simulink library "Pump_Lib"  (R2014a)
settings: Solver=ode45  StartTime=0.0  StopTime=10.0  RelTol=1e-3
undefined symbols (not defined in the file): APN_Param
libraries: Pump_Lib x3, powerlib x3
Description:
  | Copyright 2014 The MathWorks, Inc.
settings Model: Creator=smiller  LastModifiedBy=psanghvi

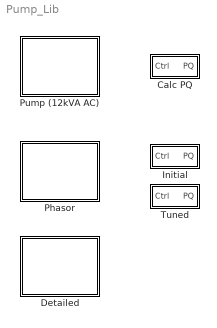
== system Pump_Lib ==
  Calc PQ : Subsystem  BlockChoice=Initial
      settings: TemplateBlock=self  MemberBlocks=Initial,Tuned
  Detailed : Subsystem
      mask Display: image(imread('PumpAC_Detailed_IMAGE.jpg'));
  Initial : Subsystem
  Phasor : Subsystem
      mask Display: image(imread('PumpAC_Phasor_IMAGE.jpg'));
  Pump (12kVA AC) : Subsystem  BlockChoice=Detailed
      settings: TemplateBlock=self  MemberBlocks=Detailed,Phasor
  Tuned : Subsystem

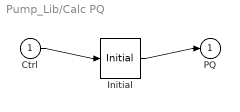
== system Pump_Lib/Calc PQ ==
  Ctrl : Inport
  Initial : Pump_Lib/Initial
  PQ : Outport
  wires:
  Ctrl/1 -> Initial/1
  Initial/1 -> PQ/1

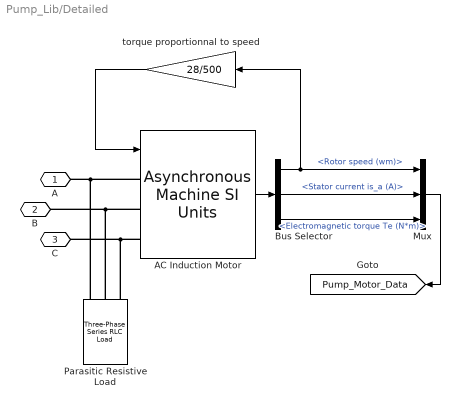
== system Pump_Lib/Detailed ==
  AC Induction Motor : powerlib/Machines/Asynchronous Machine SI Units  PresetModel=No  MechanicalLoad=Torque Tm  ShowDetailedParameters=on  RotorType=Squirrel-cage  ReferenceFrame=Rotor  Units=SI  MeasurementBus=off  NominalParameters=[12e3 200 400]  Stator=[0.2761 0.002191/10]  Rotor=[0.16 0.002191/10]  Cage1=[ 0.022 0.226/377]  Cage2=[ 0.022 0.226/377]  Lm=0.07614  Mechanical=[0.01 0 8]  PolePairs=8  InitialConditions=[0 0 0.850924 0.850924 0.850924 -89.9171 -209.917 30.0829]*0+[0,0 0,0,0 0,0,0]  SimulateSaturation=off  Saturation=[14.03593122, 27.81365428, 53.79336849, 72.68890987, 97.98006896, 148.6815601, 215.7428561, 302.9841135, 428.7778367 ; 230, 322, 414, 460, 506, 552, 598, 644, 690]  LoadFlowParameters=0  TsPowergui=0  TsBlock=-1  IterativeModel=Forward Euler  Pmec=0
  Bus Selector : BusSelector  OutputSignals=Mechanical.Rotor speed (wm),Stator measurements.Stator current is_a (A),Mechanical.Electromagnetic torque Te (N*m)
  Mux : Mux  Inputs=3
  Parasitic Resistive Load : powerlib/Elements/Three-Phase Series RLC Load  LConnTagsString=A|B|C  Configuration=Y (grounded)  NominalVoltage=200  NominalFrequency=400  ActivePower=1200  InductivePower=0  CapacitivePower=0  Measurements=None  LoadType=constant Z
  torque proportionnal to speed : Gain  Gain=28/500
  A : PMIOPort  Port=1  Side=Left
  B : PMIOPort  Port=2  Side=Left
  C : PMIOPort  Port=3  Side=Left
  tag scope: Pump_Motor_Data=global
  wires:
  Bus Selector/3 -> Mux/3  "<Electromagnetic torque Te (N*m)>"
  Bus Selector/2 -> Mux/2  "<Stator current is_a (A)>"
  torque proportionnal to speed/1 -> AC Induction Motor/1
  Bus Selector/1 -> Mux/1, torque proportionnal to speed/1  "<Rotor speed (wm)>"
  AC Induction Motor/1 -> Bus Selector/1
  Mux/1 -> [Pump_Motor_Data]
  connections:
  AC Induction Motor/LConn3 -- Parasitic Resistive Load/LConn3 -- C/RConn1
  AC Induction Motor/LConn1 -- Parasitic Resistive Load/LConn1 -- A/RConn1
  AC Induction Motor/LConn2 -- Parasitic Resistive Load/LConn2 -- B/RConn1

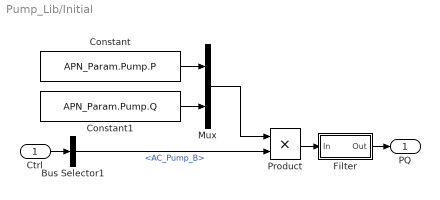
== system Pump_Lib/Initial ==
  Ctrl : Inport
  Bus Selector1 : BusSelector  OutputSignals=AC_Pump_B
  Constant : Constant  Value=APN_Param.Pump.P
  Constant1 : Constant  Value=APN_Param.Pump.Q
  Filter : Subsystem  mask(First-order lag supporting vector signals){b=1e-2, x_initial=[APN_Param.Pump.P APN_Param.Pump.Q]*0}
      mask prompts: b "Filter time constant"; x_initial "Initial output"
      mask help: Models a lag of the form 1/(b*s+1) where s is the Laplace operator.
  Mux : Mux  Inputs=2
  Product : Product
  PQ : Outport
  wires:
  Product/1 -> Filter/1(In)
  Filter/1(Out) -> PQ/1
  Bus Selector1/1 -> Product/2  "<AC_Pump_B>"
  Mux/1 -> Product/1
  Ctrl/1 -> Bus Selector1/1
  Constant/1 -> Mux/1
  Constant1/1 -> Mux/2

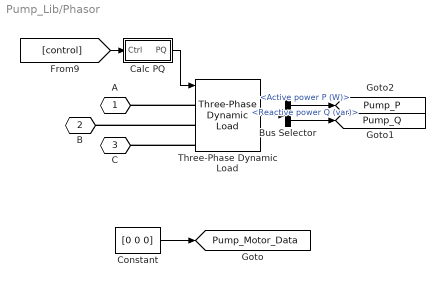
== system Pump_Lib/Phasor ==
  Bus Selector : BusSelector  OutputSignals=Active power P (W),Reactive power Q (var)
  Calc PQ : Subsystem  BlockChoice=Initial
      settings: AttributesFormatString=%<BlockChoice>  TemplateBlock=Pump_Lib/Calc PQ  MemberBlocks=Initial,Tuned
  Constant : Constant  Value=[0 0 0]
  Three-Phase Dynamic Load : powerlib/Elements/Three-Phase Dynamic Load  NominalVoltage=[ 500e3 400 ]  ActiveReactivePowers=[APN_Param.Pump.P APN_Param.Pump.Q]  PositiveSequence=[0.0004 0]  ExternalControl=on  NpNq=[1.3 2]  TimeConstants="[0  0  0  0]"  MinimumVoltage=0.7  LoadFlowParameters=[4 0 0 0 0]
  A : PMIOPort  Port=1  Side=Left
  B : PMIOPort  Port=2  Side=Left
  C : PMIOPort  Port=3  Side=Left
  tag scope: Pump_Motor_Data=global, Pump_P=global, Pump_Q=global
  wires:
  Bus Selector/1 -> [Pump_P]  "<Active power P (W)>"
  Three-Phase Dynamic Load/1 -> Bus Selector/1
  Bus Selector/2 -> [Pump_Q]  "<Reactive power Q (var)>"
  [control] -> Calc PQ/1(Ctrl)
  Calc PQ/1(PQ) -> Three-Phase Dynamic Load/1
  Constant/1 -> [Pump_Motor_Data]
  connections:
  Three-Phase Dynamic Load/LConn3 -- C/RConn1
  Three-Phase Dynamic Load/LConn2 -- B/RConn1
  Three-Phase Dynamic Load/LConn1 -- A/RConn1

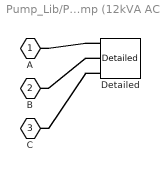
== system Pump_Lib/Pump (12kVA AC) ==
  Detailed : Pump_Lib/Detailed  SystemSampleTime=-1
  A : PMIOPort  Port=1  Side=Left
  B : PMIOPort  Port=2  Side=Left
  C : PMIOPort  Port=3  Side=Left
  connections:
  Detailed/LConn1 -- A/RConn1
  Detailed/LConn2 -- B/RConn1
  Detailed/LConn3 -- C/RConn1

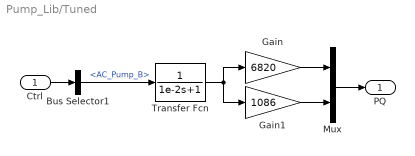
== system Pump_Lib/Tuned ==
  Ctrl : Inport
  Bus Selector1 : BusSelector  OutputSignals=AC_Pump_B
  Gain : Gain  Gain=6820
  Gain1 : Gain  Gain=1086
  Mux : Mux  Inputs=2
  Transfer Fcn : TransferFcn  Denominator=[1e-2 1]
  PQ : Outport
  wires:
  Ctrl/1 -> Bus Selector1/1
  Bus Selector1/1 -> Transfer Fcn/1  "<AC_Pump_B>"
  Gain1/1 -> Mux/2
  Gain/1 -> Mux/1
  Mux/1 -> PQ/1
  Transfer Fcn/1 -> Gain/1, Gain1/1

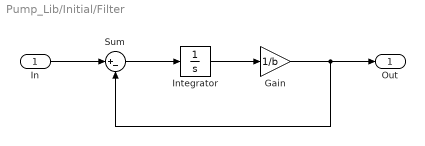
== system Pump_Lib/Initial/Filter ==
  In : Inport
  Gain : Gain  Gain=1/b
  Integrator : Integrator  InitialCondition=x_initial
  Sum : Sum  Inputs=|+-  SaturateOnIntegerOverflow=on  InputSameDT=on  OutDataTypeStr=Inherit: Same as first input
  Out : Outport
  wires:
  Gain/1 -> Out/1, Sum/2
  Integrator/1 -> Gain/1
  In/1 -> Sum/1
  Sum/1 -> Integrator/1

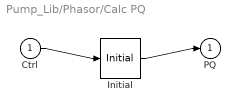
== system Pump_Lib/Phasor/Calc PQ ==
  Ctrl : Inport
  Initial : Pump_Lib/Initial
  PQ : Outport
  wires:
  Ctrl/1 -> Initial/1
  Initial/1 -> PQ/1
